simulink library "halin"  (R2021b)
settings: Solver=VariableStepAuto  StartTime=0.0  StopTime=10.0  RelTol=1e-3
undefined symbols (not defined in the file): KHAL_CAN1ABM1E2E_flg, KHAL_CAN1EPB1E2E_flg, KHAL_CAN1EPS1E2E_flg, KHAL_CAN1ESC1E2E_flg, KHAL_CAN1ESC5E2E_flg, KHAL_CAN3BMS1E2E_flg, KHAL_CAN3BMS6E2E_flg, KHAL_CAN3CCU1E2E_flg, KHAL_CAN3CCU2E2E_flg, KHAL_CAN3MCUNF1E2E_flg, KHAL_CAN3MCUNR1E2E_flg, KHAL_CAN3Shifter1E2E_flg, KHAL_CAN3Shifter2E2E_flg, KHAL_CAN6FCM2E2E_flg, KHAL_CAN6FCM4E2E_flg, TRUE
libraries: simulink x645, FVT_lib x212, hcu_lib x59
(part 9 of 23)

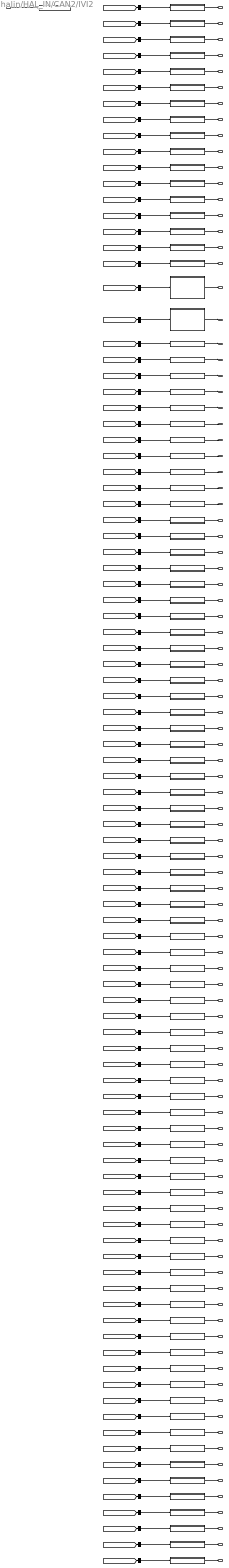
== system halin/HAL_IN/CAN2/IVI2 ==
  DT_CAN2_SG_IVI2 : Inport
  ACChgCurSet : Subsystem
  AVMErrSTA : Subsystem
  AVMOFFRecButt : Subsystem
  AVMParkingmode : Subsystem
  AVMparkingcancel : Subsystem
  AVMparkingexcute : Subsystem
  ApproachUnlockSW : Subsystem
  CAASSw : Subsystem
  CDLLockButt : Subsystem
  CDLUnlockButt : Subsystem
  DSEATantiset : Subsystem
  DSEATentryfunset : Subsystem
  DSEATventreq : Subsystem
  Distanceunit : Subsystem
  ESCSWCmd : Subsystem
  FSOffSw : Subsystem
  FollowMeSW : Subsystem
  GPSLAT : Subsystem
  GPSLONG : Subsystem
  HeadLampSW : Subsystem
  HoodLatchSW : Subsystem
  IVIACCAdaptiveSta : Subsystem
  IVIAirIntZ3Cmd : Subsystem
  IVIChargePortSWSta : Subsystem
  IVICreepSWReq : Subsystem
  IVIDSEATFroEdgeHeightCmd : Subsystem
  IVIDSEATHeaterCmd : Subsystem
  IVIDSEATHeightCmd : Subsystem
  IVIDSEATMemory1Sta : Subsystem
  IVIDSEATMemory2Sta : Subsystem
  IVIDSEATMemoryOPTCLSSta : Subsystem
  IVIDSEATReclineCmd : Subsystem
  IVIDSEATSlideCmd : Subsystem
  IVIFGSAirIntCmd : Subsystem
  IVIFGSChCmd : Subsystem
  IVIIONSWCmd : Subsystem
  IVIISAOffsetSpd : Subsystem
  IVINightModeSta : Subsystem
  IVIPSEATHeaterCmd : Subsystem
  IVIPSEATReclineCmd : Subsystem
  IVIPSEATSlideCmd : Subsystem
  IVIPTGModeSW : Subsystem
  IVIPTGOpenHeight : Subsystem
  IVIPTGStaSW : Subsystem
  IVIPTGUSStaSW : Subsystem
  IVIPWModeReq : Subsystem
  IVIPwrLockSW : Subsystem
  IVIPwroffreq : Subsystem
  IVIRRDefReq : Subsystem
  IVIReqV2L : Subsystem
  IVISWCRUndefinedSta : Subsystem
  IVIScreen : Subsystem
  IVIStartChgreq : Subsystem
  IVIStatus : Subsystem
  IVIStopChgreq : Subsystem
  IVITrailerCheckReqSta : Subsystem
  IVITrailerModeSWSta : Subsystem
  IVITriggerreq : Subsystem
  IVIUnlockChgreq : Subsystem
  IVIWIMAINSW : Subsystem
  LDrvControlCommand : Subsystem
  LPasControlCommand : Subsystem
  LRLDControlCommand : Subsystem
  LRRDControlCommand : Subsystem
  LightShowStartReq : Subsystem
  LightShowStopReq : Subsystem
  MFRDNBrightReq : Subsystem
  OFFACMODE : Subsystem
  PSEATventreq : Subsystem
  PerdV2L : Subsystem
  RFogLampSW : Subsystem
  RollModeSWCmd : Subsystem
  RoomLampMode : Subsystem
  SOCADJBUTT : Subsystem
  SOCLimitSet : Subsystem
  SOCV2LLimit : Subsystem
  SchedChgStart : Subsystem
  SchedChgStop : Subsystem
  SchedChgbutt : Subsystem
  SchedChglimit : Subsystem
  SchedChgwake : Subsystem
  SenstivityPosition : Subsystem
  SetUnlockSingle : Subsystem
  TCSSWCmd : Subsystem
  TPMSCaliButt : Subsystem
  TPMSResButt : Subsystem
  TurnSwTimeSet : Subsystem
  WalkawayLockSW : Subsystem
  WlcmLightMode : Subsystem
  bus_selector : BusSelector  OutputSignals=CAN2_AC_Chg_Cur_Set
  bus_selector1 : BusSelector  OutputSignals=CAN2_AVM_Err_STA
  bus_selector10 : BusSelector  OutputSignals=CAN2_DSEAT_anti_set
  bus_selector11 : BusSelector  OutputSignals=CAN2_DSEAT_entryfun_set
  bus_selector12 : BusSelector  OutputSignals=CAN2_DSEAT_vent_req
  bus_selector13 : BusSelector  OutputSignals=CAN2_Distance_unit
  bus_selector14 : BusSelector  OutputSignals=CAN2_ESC_SW_Cmd
  bus_selector15 : BusSelector  OutputSignals=CAN2_FS_Off_Sw
  bus_selector16 : BusSelector  OutputSignals=CAN2_FollowMeSW
  bus_selector17 : BusSelector  OutputSignals=CAN2_GPS_LAT
  bus_selector18 : BusSelector  OutputSignals=CAN2_GPS_LONG
  bus_selector19 : BusSelector  OutputSignals=CAN2_HeadLampSW
  bus_selector2 : BusSelector  OutputSignals=CAN2_AVM_OFF_Rec_Butt
  bus_selector20 : BusSelector  OutputSignals=CAN2_Hood_Latch_SW
  bus_selector21 : BusSelector  OutputSignals=CAN2_IVI_ACC_Adaptive_Sta
  bus_selector22 : BusSelector  OutputSignals=CAN2_IVI_AirIntZ3_Cmd
  bus_selector23 : BusSelector  OutputSignals=CAN2_IVI_ChargePortSW_Sta
  bus_selector24 : BusSelector  OutputSignals=CAN2_IVI_CreepSW_Req
  bus_selector25 : BusSelector  OutputSignals=CAN2_IVI_DSEATHeater_Cmd
  bus_selector26 : BusSelector  OutputSignals=CAN2_IVI_DSEAT_FroEdge_Height_Cmd
  bus_selector27 : BusSelector  OutputSignals=CAN2_IVI_DSEAT_Height_Cmd
  bus_selector28 : BusSelector  OutputSignals=CAN2_IVI_DSEAT_Memory1_Sta
  bus_selector29 : BusSelector  OutputSignals=CAN2_IVI_DSEAT_Memory2_Sta
  bus_selector3 : BusSelector  OutputSignals=CAN2_AVM_Parking_mode
  bus_selector30 : BusSelector  OutputSignals=CAN2_IVI_DSEAT_Memory_OPTCLS_Sta
  bus_selector31 : BusSelector  OutputSignals=CAN2_IVI_DSEAT_Recline_Cmd
  bus_selector32 : BusSelector  OutputSignals=CAN2_IVI_DSEAT_Slide_Cmd
  bus_selector33 : BusSelector  OutputSignals=CAN2_IVI_FGSAirInt_Cmd
  bus_selector34 : BusSelector  OutputSignals=CAN2_IVI_FGSCh_Cmd
  bus_selector35 : BusSelector  OutputSignals=CAN2_IVI_IONSW_Cmd
  bus_selector36 : BusSelector  OutputSignals=CAN2_IVI_ISA_OffsetSpd
  bus_selector37 : BusSelector  OutputSignals=CAN2_IVI_Night_Mode_Sta
  bus_selector38 : BusSelector  OutputSignals=CAN2_IVI_PSEATHeater_Cmd
  bus_selector39 : BusSelector  OutputSignals=CAN2_IVI_PSEAT_Recline_Cmd
  bus_selector4 : BusSelector  OutputSignals=CAN2_AVM_parking_cancel
  bus_selector40 : BusSelector  OutputSignals=CAN2_IVI_PSEAT_Slide_Cmd
  bus_selector41 : BusSelector  OutputSignals=CAN2_IVI_PTG_Mode_SW
  bus_selector42 : BusSelector  OutputSignals=CAN2_IVI_PTG_Open_Height
  bus_selector43 : BusSelector  OutputSignals=CAN2_IVI_PTG_Sta_SW
  bus_selector44 : BusSelector  OutputSignals=CAN2_IVI_PTG_USSta_SW
  bus_selector45 : BusSelector  OutputSignals=CAN2_IVI_PW_Mode_Req
  bus_selector46 : BusSelector  OutputSignals=CAN2_IVI_PwrLockSW
  bus_selector47 : BusSelector  OutputSignals=CAN2_IVI_Pwroff_req
  bus_selector48 : BusSelector  OutputSignals=CAN2_IVI_RR_Def_Req
  bus_selector49 : BusSelector  OutputSignals=CAN2_IVI_Req_V2L
  bus_selector5 : BusSelector  OutputSignals=CAN2_AVM_parking_excute
  bus_selector50 : BusSelector  OutputSignals=CAN2_IVI_SWC_RUndefined_Sta
  bus_selector51 : BusSelector  OutputSignals=CAN2_IVI_Screen
  bus_selector52 : BusSelector  OutputSignals=CAN2_IVI_Start_Chg_req
  bus_selector53 : BusSelector  OutputSignals=CAN2_IVI_Status
  bus_selector54 : BusSelector  OutputSignals=CAN2_IVI_Stop_Chg_req
  bus_selector55 : BusSelector  OutputSignals=CAN2_IVI_TrailerCheckReq_Sta
  bus_selector56 : BusSelector  OutputSignals=CAN2_IVI_TrailerModeSW_Sta
  bus_selector57 : BusSelector  OutputSignals=CAN2_IVI_Trigger_req
  bus_selector58 : BusSelector  OutputSignals=CAN2_IVI_Unlock_Chg_req
  bus_selector59 : BusSelector  OutputSignals=CAN2_IVI_WI_MAIN_SW
  bus_selector6 : BusSelector  OutputSignals=CAN2_Approach_Unlock_SW
  bus_selector60 : BusSelector  OutputSignals=CAN2_L_Drv_ControlCommand
  bus_selector61 : BusSelector  OutputSignals=CAN2_L_Pas_ControlCommand
  bus_selector62 : BusSelector  OutputSignals=CAN2_L_RLD_ControlCommand
  bus_selector63 : BusSelector  OutputSignals=CAN2_L_RRD_ControlCommand
  bus_selector64 : BusSelector  OutputSignals=CAN2_Light_ShowStart_Req
  bus_selector65 : BusSelector  OutputSignals=CAN2_Light_ShowStop_Req
  bus_selector66 : BusSelector  OutputSignals=CAN2_MFRD_N_Bright_Req
  bus_selector67 : BusSelector  OutputSignals=CAN2_OFF_AC_MODE
  bus_selector68 : BusSelector  OutputSignals=CAN2_PSEAT_vent_req
  bus_selector69 : BusSelector  OutputSignals=CAN2_Perd_V2L
  bus_selector7 : BusSelector  OutputSignals=CAN2_CAAS_Sw
  bus_selector70 : BusSelector  OutputSignals=CAN2_RFogLampSW
  bus_selector71 : BusSelector  OutputSignals=CAN2_Roll_Mode_SW_Cmd
  bus_selector72 : BusSelector  OutputSignals=CAN2_RoomLampMode
  bus_selector73 : BusSelector  OutputSignals=CAN2_SOC_ADJ_BUTT
  bus_selector74 : BusSelector  OutputSignals=CAN2_SOC_Limit_Set
  bus_selector75 : BusSelector  OutputSignals=CAN2_SOC_V2LLimit
  bus_selector76 : BusSelector  OutputSignals=CAN2_Sched_Chg_Start
  bus_selector77 : BusSelector  OutputSignals=CAN2_Sched_Chg_Stop
  bus_selector78 : BusSelector  OutputSignals=CAN2_Sched_Chg_butt
  bus_selector79 : BusSelector  OutputSignals=CAN2_Sched_Chg_limit
  bus_selector8 : BusSelector  OutputSignals=CAN2_CDL_Lock_Butt
  bus_selector80 : BusSelector  OutputSignals=CAN2_Sched_Chg_wake
  bus_selector81 : BusSelector  OutputSignals=CAN2_SenstivityPosition
  bus_selector82 : BusSelector  OutputSignals=CAN2_SetUnlockSingle
  bus_selector83 : BusSelector  OutputSignals=CAN2_TCS_SW_Cmd
  bus_selector84 : BusSelector  OutputSignals=CAN2_TPMS_Cali_Butt
  bus_selector85 : BusSelector  OutputSignals=CAN2_TPMS_Res_Butt
  bus_selector86 : BusSelector  OutputSignals=CAN2_TurnSwTimeSet
  bus_selector87 : BusSelector  OutputSignals=CAN2_Walkaway_Lock_SW
  bus_selector88 : BusSelector  OutputSignals=CAN2_WlcmLight_Mode
  bus_selector89 : BusSelector  OutputSignals=CAN2_sigAirIntenZon1Req
  bus_selector9 : BusSelector  OutputSignals=CAN2_CDL_Unlock_Butt
  bus_selector90 : BusSelector  OutputSignals=CAN2_sigDfrstReq
  bus_selector91 : BusSelector  OutputSignals=CAN2_sigFaceReq
  bus_selector92 : BusSelector  OutputSignals=CAN2_sigFootReq
  bus_selector93 : BusSelector  OutputSignals=CAN2_sigRecircReq
  bus_selector94 : BusSelector  OutputSignals=CAN2_sigSetTempZon1Req
  bus_selector95 : BusSelector  OutputSignals=CAN2_sigSetTempZon2Req
  sigAirIntenZon1Req : Subsystem
  sigDfrstReq : Subsystem
  sigFaceReq : Subsystem
  sigFootReq : Subsystem
  sigRecircReq : Subsystem
  sigSetTempZon1Req : Subsystem
  sigSetTempZon2Req : Subsystem
  VHAL_ACChgCurSet_A : Outport
  VHAL_AVMErrSTA_flg : Outport  Port=2
  VHAL_AVMOFFRecButt_flg : Outport  Port=3
  VHAL_AVMParkingmode_enum : Outport  Port=4
  VHAL_AVMparkingcancel_enum : Outport  Port=5
  VHAL_AVMparkingexcute_enum : Outport  Port=6
  VHAL_ApproachUnlockSW_flg : Outport  Port=7
  VHAL_CAASSw_enum : Outport  Port=8
  VHAL_CDLLockButt_flg : Outport  Port=9
  VHAL_CDLUnlockButt_flg : Outport  Port=10
  VHAL_DSEATantiset_flg : Outport  Port=11
  VHAL_DSEATentryfunset_flg : Outport  Port=12
  VHAL_DSEATventreq_enum : Outport  Port=13
  VHAL_Distanceunit_flg : Outport  Port=14
  VHAL_ESCSWCmd_enum : Outport  Port=15
  VHAL_FSOffSw_enum : Outport  Port=16
  VHAL_FollowMeSW_flg : Outport  Port=17
  VHAL_GPSLAT_s : Outport  Port=18
  VHAL_GPSLONG_enum : Outport  Port=19
  VHAL_HeadLampSW_enum : Outport  Port=20
  VHAL_HoodLatchSW_enum : Outport  Port=21
  VHAL_IVIACCAdaptiveSta_flg : Outport  Port=22
  VHAL_IVIAirIntZ3Cmd_enum : Outport  Port=23
  VHAL_IVIChargePortSWSta_flg : Outport  Port=24
  VHAL_IVICreepSWReq_flg : Outport  Port=25
  VHAL_IVIDSEATHeaterCmd_enum : Outport  Port=26
  VHAL_IVIDSEATFroEdgeHeightCmd_enum : Outport  Port=27
  VHAL_IVIDSEATHeightCmd_enum : Outport  Port=28
  VHAL_IVIDSEATMemory1Sta_flg : Outport  Port=29
  VHAL_IVIDSEATMemory2Sta_flg : Outport  Port=30
  VHAL_IVIDSEATMemoryOPTCLSSta_flg : Outport  Port=31
  VHAL_IVIDSEATReclineCmd_enum : Outport  Port=32
  VHAL_IVIDSEATSlideCmd_enum : Outport  Port=33
  VHAL_IVIFGSAirIntCmd_enum : Outport  Port=34
  VHAL_IVIFGSChCmd_enum : Outport  Port=35
  VHAL_IVIIONSWCmd_flg : Outport  Port=36
  VHAL_IVIISAOffsetSpd_enum : Outport  Port=37
  VHAL_IVINightModeSta_flg : Outport  Port=38
  VHAL_IVIPSEATHeaterCmd_enum : Outport  Port=39
  VHAL_IVIPSEATReclineCmd_enum : Outport  Port=40
  VHAL_IVIPSEATSlideCmd_enum : Outport  Port=41
  VHAL_IVIPTGModeSW_enum : Outport  Port=42
  VHAL_IVIPTGOpenHeight_enum : Outport  Port=43
  VHAL_IVIPTGStaSW_enum : Outport  Port=44
  VHAL_IVIPTGUSStaSW_flg : Outport  Port=45
  VHAL_IVIPWModeReq_enum : Outport  Port=46
  VHAL_IVIPwrLockSW_enum : Outport  Port=47
  VHAL_IVIPwroffreq_flg : Outport  Port=48
  VHAL_IVIRRDefReq_flg : Outport  Port=49
  VHAL_IVIReqV2L_enum : Outport  Port=50
  VHAL_IVISWCRUndefinedSta_enum : Outport  Port=51
  VHAL_IVIScreen_enum : Outport  Port=52
  VHAL_IVIStartChgreq_flg : Outport  Port=53
  VHAL_IVIStatus_flg : Outport  Port=54
  VHAL_IVIStopChgreq_flg : Outport  Port=55
  VHAL_IVITrailerCheckReqSta_flg : Outport  Port=56
  VHAL_IVITrailerModeSWSta_flg : Outport  Port=57
  VHAL_IVITriggerreq_flg : Outport  Port=58
  VHAL_IVIUnlockChgreq_flg : Outport  Port=59
  VHAL_IVIWIMAINSW_flg : Outport  Port=60
  VHAL_LDrvControlCommand_pct : Outport  Port=61
  VHAL_LPasControlCommand_pct : Outport  Port=62
  VHAL_LRLDControlCommand_pct : Outport  Port=63
  VHAL_LRRDControlCommand_pct : Outport  Port=64
  VHAL_LightShowStartReq_flg : Outport  Port=65
  VHAL_LightShowStopReq_flg : Outport  Port=66
  VHAL_MFRDNBrightReq_pct : Outport  Port=67
  VHAL_OFFACMODE_enum : Outport  Port=68
  VHAL_PSEATventreq_enum : Outport  Port=69
  VHAL_PerdV2L_enum : Outport  Port=70
  VHAL_RFogLampSW_flg : Outport  Port=71
  VHAL_RollModeSWCmd_enum : Outport  Port=72
  VHAL_RoomLampMode_flg : Outport  Port=73
  VHAL_SOCADJBUTT_flg : Outport  Port=74
  VHAL_SOCLimitSet_pct : Outport  Port=75
  VHAL_SOCV2LLimit_pct : Outport  Port=76
  VHAL_SchedChgStart_flg : Outport  Port=77
  VHAL_SchedChgStop_flg : Outport  Port=78
  VHAL_SchedChgbutt_flg : Outport  Port=79
  VHAL_SchedChglimit_pct : Outport  Port=80
  VHAL_SchedChgwake_flg : Outport  Port=81
  VHAL_SenstivityPosition_enum : Outport  Port=82
  VHAL_SetUnlockSingle_flg : Outport  Port=83
  VHAL_TCSSWCmd_enum : Outport  Port=84
  VHAL_TPMSCaliButt_flg : Outport  Port=85
  VHAL_TPMSResButt_flg : Outport  Port=86
  VHAL_TurnSwTimeSet_enum : Outport  Port=87
  VHAL_WalkawayLockSW_flg : Outport  Port=88
  VHAL_WlcmLightMode_enum : Outport  Port=89
  VHAL_sigAirIntenZon1Req_enum : Outport  Port=90
  VHAL_sigDfrstReq_flg : Outport  Port=91
  VHAL_sigFaceReq_flg : Outport  Port=92
  VHAL_sigFootReq_flg : Outport  Port=93
  VHAL_sigRecircReq_flg : Outport  Port=94
  VHAL_sigSetTempZon1Req_C : Outport  Port=95
  VHAL_sigSetTempZon2Req_C : Outport  Port=96
  wires:
  DT_CAN2_SG_IVI2/1 -> [DT_CAN2_SG_IVI2]
  [DT_CAN2_SG_IVI2] -> bus_selector/1
  bus_selector/1 -> ACChgCurSet/1(AC_Chg_Cur_Set)  "<CAN2_AC_Chg_Cur_Set>"
  ACChgCurSet/1(VHAL_ACChgCurSet_A) -> VHAL_ACChgCurSet_A/1
  [DT_CAN2_SG_IVI2] -> bus_selector1/1
  bus_selector1/1 -> AVMErrSTA/1(AVM_Err_STA)  "<CAN2_AVM_Err_STA>"
  AVMErrSTA/1(VHAL_AVMErrSTA_flg) -> VHAL_AVMErrSTA_flg/1
  [DT_CAN2_SG_IVI2] -> bus_selector2/1
  bus_selector2/1 -> AVMOFFRecButt/1(AVM_OFF_Rec_Butt)  "<CAN2_AVM_OFF_Rec_Butt>"
  AVMOFFRecButt/1(VHAL_AVMOFFRecButt_flg) -> VHAL_AVMOFFRecButt_flg/1
  [DT_CAN2_SG_IVI2] -> bus_selector3/1
  bus_selector3/1 -> AVMParkingmode/1(AVM_Parking_mode)  "<CAN2_AVM_Parking_mode>"
  AVMParkingmode/1(VHAL_AVMParkingmode_enum) -> VHAL_AVMParkingmode_enum/1
  [DT_CAN2_SG_IVI2] -> bus_selector4/1
  bus_selector4/1 -> AVMparkingcancel/1(AVM_parking_cancel)  "<CAN2_AVM_parking_cancel>"
  AVMparkingcancel/1(VHAL_AVMparkingcancel_enum) -> VHAL_AVMparkingcancel_enum/1
  [DT_CAN2_SG_IVI2] -> bus_selector5/1
  bus_selector5/1 -> AVMparkingexcute/1(AVM_parking_excute)  "<CAN2_AVM_parking_excute>"
  AVMparkingexcute/1(VHAL_AVMparkingexcute_enum) -> VHAL_AVMparkingexcute_enum/1
  [DT_CAN2_SG_IVI2] -> bus_selector6/1
  bus_selector6/1 -> ApproachUnlockSW/1(Approach_Unlock_SW)  "<CAN2_Approach_Unlock_SW>"
  ApproachUnlockSW/1(VHAL_ApproachUnlockSW_flg) -> VHAL_ApproachUnlockSW_flg/1
  [DT_CAN2_SG_IVI2] -> bus_selector7/1
  bus_selector7/1 -> CAASSw/1(CAAS_Sw)  "<CAN2_CAAS_Sw>"
  CAASSw/1(VHAL_CAASSw_enum) -> VHAL_CAASSw_enum/1
  [DT_CAN2_SG_IVI2] -> bus_selector8/1
  bus_selector8/1 -> CDLLockButt/1(CDL_Lock_Butt)  "<CAN2_CDL_Lock_Butt>"
  CDLLockButt/1(VHAL_CDLLockButt_flg) -> VHAL_CDLLockButt_flg/1
  [DT_CAN2_SG_IVI2] -> bus_selector9/1
  bus_selector9/1 -> CDLUnlockButt/1(CDL_Unlock_Butt)  "<CAN2_CDL_Unlock_Butt>"
  CDLUnlockButt/1(VHAL_CDLUnlockButt_flg) -> VHAL_CDLUnlockButt_flg/1
  [DT_CAN2_SG_IVI2] -> bus_selector10/1
  bus_selector10/1 -> DSEATantiset/1(DSEAT_anti_set)  "<CAN2_DSEAT_anti_set>"
  DSEATantiset/1(VHAL_DSEATantiset_flg) -> VHAL_DSEATantiset_flg/1
  [DT_CAN2_SG_IVI2] -> bus_selector11/1
  bus_selector11/1 -> DSEATentryfunset/1(DSEAT_entryfun_set)  "<CAN2_DSEAT_entryfun_set>"
  DSEATentryfunset/1(VHAL_DSEATentryfunset_flg) -> VHAL_DSEATentryfunset_flg/1
  [DT_CAN2_SG_IVI2] -> bus_selector12/1
  bus_selector12/1 -> DSEATventreq/1(DSEAT_vent_req)  "<CAN2_DSEAT_vent_req>"
  DSEATventreq/1(VHAL_DSEATventreq_enum) -> VHAL_DSEATventreq_enum/1
  [DT_CAN2_SG_IVI2] -> bus_selector13/1
  bus_selector13/1 -> Distanceunit/1(Distance_unit)  "<CAN2_Distance_unit>"
  Distanceunit/1(VHAL_Distanceunit_flg) -> VHAL_Distanceunit_flg/1
  [DT_CAN2_SG_IVI2] -> bus_selector14/1
  bus_selector14/1 -> ESCSWCmd/1(ESC_SW_Cmd)  "<CAN2_ESC_SW_Cmd>"
  ESCSWCmd/1(VHAL_ESCSWCmd_enum) -> VHAL_ESCSWCmd_enum/1
  [DT_CAN2_SG_IVI2] -> bus_selector15/1
  bus_selector15/1 -> FSOffSw/1(FS_Off_Sw)  "<CAN2_FS_Off_Sw>"
  FSOffSw/1(VHAL_FSOffSw_enum) -> VHAL_FSOffSw_enum/1
  [DT_CAN2_SG_IVI2] -> bus_selector16/1
  bus_selector16/1 -> FollowMeSW/1(FollowMeSW)  "<CAN2_FollowMeSW>"
  FollowMeSW/1(VHAL_FollowMeSW_flg) -> VHAL_FollowMeSW_flg/1
  [DT_CAN2_SG_IVI2] -> bus_selector17/1
  bus_selector17/1 -> GPSLAT/1(GPS_LAT)  "<CAN2_GPS_LAT>"
  GPSLAT/1(VHAL_GPSLAT_s) -> VHAL_GPSLAT_s/1
  [DT_CAN2_SG_IVI2] -> bus_selector18/1
  bus_selector18/1 -> GPSLONG/1(GPS_LONG)  "<CAN2_GPS_LONG>"
  GPSLONG/1(VHAL_GPSLONG_enum) -> VHAL_GPSLONG_enum/1
  [DT_CAN2_SG_IVI2] -> bus_selector19/1
  bus_selector19/1 -> HeadLampSW/1(HeadLampSW)  "<CAN2_HeadLampSW>"
  HeadLampSW/1(VHAL_HeadLampSW_enum) -> VHAL_HeadLampSW_enum/1
  [DT_CAN2_SG_IVI2] -> bus_selector20/1
  bus_selector20/1 -> HoodLatchSW/1(Hood_Latch_SW)  "<CAN2_Hood_Latch_SW>"
  HoodLatchSW/1(VHAL_HoodLatchSW_enum) -> VHAL_HoodLatchSW_enum/1
  [DT_CAN2_SG_IVI2] -> bus_selector21/1
  bus_selector21/1 -> IVIACCAdaptiveSta/1(IVI_ACC_Adaptive_Sta)  "<CAN2_IVI_ACC_Adaptive_Sta>"
  IVIACCAdaptiveSta/1(VHAL_IVIACCAdaptiveSta_flg) -> VHAL_IVIACCAdaptiveSta_flg/1
  [DT_CAN2_SG_IVI2] -> bus_selector22/1
  bus_selector22/1 -> IVIAirIntZ3Cmd/1(IVI_AirIntZ3_Cmd)  "<CAN2_IVI_AirIntZ3_Cmd>"
  IVIAirIntZ3Cmd/1(VHAL_IVIAirIntZ3Cmd_enum) -> VHAL_IVIAirIntZ3Cmd_enum/1
  [DT_CAN2_SG_IVI2] -> bus_selector23/1
  bus_selector23/1 -> IVIChargePortSWSta/1(IVI_ChargePortSW_Sta)  "<CAN2_IVI_ChargePortSW_Sta>"
  IVIChargePortSWSta/1(VHAL_IVIChargePortSWSta_flg) -> VHAL_IVIChargePortSWSta_flg/1
  [DT_CAN2_SG_IVI2] -> bus_selector24/1
  bus_selector24/1 -> IVICreepSWReq/1(IVI_CreepSW_Req)  "<CAN2_IVI_CreepSW_Req>"
  IVICreepSWReq/1(VHAL_IVICreepSWReq_flg) -> VHAL_IVICreepSWReq_flg/1
  [DT_CAN2_SG_IVI2] -> bus_selector25/1
  bus_selector25/1 -> IVIDSEATHeaterCmd/1(IVI_DSEATHeater_Cmd)  "<CAN2_IVI_DSEATHeater_Cmd>"
  IVIDSEATHeaterCmd/1(VHAL_IVIDSEATHeaterCmd_enum) -> VHAL_IVIDSEATHeaterCmd_enum/1
  [DT_CAN2_SG_IVI2] -> bus_selector26/1
  bus_selector26/1 -> IVIDSEATFroEdgeHeightCmd/1(IVI_DSEAT_FroEdge_Height_Cmd)  "<CAN2_IVI_DSEAT_FroEdge_Height_Cmd>"
  IVIDSEATFroEdgeHeightCmd/1(VHAL_IVIDSEATFroEdgeHeightCmd_enum) -> VHAL_IVIDSEATFroEdgeHeightCmd_enum/1
  [DT_CAN2_SG_IVI2] -> bus_selector27/1
  bus_selector27/1 -> IVIDSEATHeightCmd/1(IVI_DSEAT_Height_Cmd)  "<CAN2_IVI_DSEAT_Height_Cmd>"
  IVIDSEATHeightCmd/1(VHAL_IVIDSEATHeightCmd_enum) -> VHAL_IVIDSEATHeightCmd_enum/1
  [DT_CAN2_SG_IVI2] -> bus_selector28/1
  bus_selector28/1 -> IVIDSEATMemory1Sta/1(IVI_DSEAT_Memory1_Sta)  "<CAN2_IVI_DSEAT_Memory1_Sta>"
  IVIDSEATMemory1Sta/1(VHAL_IVIDSEATMemory1Sta_flg) -> VHAL_IVIDSEATMemory1Sta_flg/1
  [DT_CAN2_SG_IVI2] -> bus_selector29/1
  bus_selector29/1 -> IVIDSEATMemory2Sta/1(IVI_DSEAT_Memory2_Sta)  "<CAN2_IVI_DSEAT_Memory2_Sta>"
  IVIDSEATMemory2Sta/1(VHAL_IVIDSEATMemory2Sta_flg) -> VHAL_IVIDSEATMemory2Sta_flg/1
  [DT_CAN2_SG_IVI2] -> bus_selector30/1
  bus_selector30/1 -> IVIDSEATMemoryOPTCLSSta/1(IVI_DSEAT_Memory_OPTCLS_Sta)  "<CAN2_IVI_DSEAT_Memory_OPTCLS_Sta>"
  IVIDSEATMemoryOPTCLSSta/1(VHAL_IVIDSEATMemoryOPTCLSSta_flg) -> VHAL_IVIDSEATMemoryOPTCLSSta_flg/1
  [DT_CAN2_SG_IVI2] -> bus_selector31/1
  bus_selector31/1 -> IVIDSEATReclineCmd/1(IVI_DSEAT_Recline_Cmd)  "<CAN2_IVI_DSEAT_Recline_Cmd>"
  IVIDSEATReclineCmd/1(VHAL_IVIDSEATReclineCmd_enum) -> VHAL_IVIDSEATReclineCmd_enum/1
  [DT_CAN2_SG_IVI2] -> bus_selector32/1
  bus_selector32/1 -> IVIDSEATSlideCmd/1(IVI_DSEAT_Slide_Cmd)  "<CAN2_IVI_DSEAT_Slide_Cmd>"
  IVIDSEATSlideCmd/1(VHAL_IVIDSEATSlideCmd_enum) -> VHAL_IVIDSEATSlideCmd_enum/1
  [DT_CAN2_SG_IVI2] -> bus_selector33/1
  bus_selector33/1 -> IVIFGSAirIntCmd/1(IVI_FGSAirInt_Cmd)  "<CAN2_IVI_FGSAirInt_Cmd>"
  IVIFGSAirIntCmd/1(VHAL_IVIFGSAirIntCmd_enum) -> VHAL_IVIFGSAirIntCmd_enum/1
  [DT_CAN2_SG_IVI2] -> bus_selector34/1
  bus_selector34/1 -> IVIFGSChCmd/1(IVI_FGSCh_Cmd)  "<CAN2_IVI_FGSCh_Cmd>"
  IVIFGSChCmd/1(VHAL_IVIFGSChCmd_enum) -> VHAL_IVIFGSChCmd_enum/1
  [DT_CAN2_SG_IVI2] -> bus_selector35/1
  bus_selector35/1 -> IVIIONSWCmd/1(IVI_IONSW_Cmd)  "<CAN2_IVI_IONSW_Cmd>"
  IVIIONSWCmd/1(VHAL_IVIIONSWCmd_flg) -> VHAL_IVIIONSWCmd_flg/1
  [DT_CAN2_SG_IVI2] -> bus_selector36/1
  bus_selector36/1 -> IVIISAOffsetSpd/1(IVI_ISA_OffsetSpd)  "<CAN2_IVI_ISA_OffsetSpd>"
  IVIISAOffsetSpd/1(VHAL_IVIISAOffsetSpd_enum) -> VHAL_IVIISAOffsetSpd_enum/1
  [DT_CAN2_SG_IVI2] -> bus_selector37/1
  bus_selector37/1 -> IVINightModeSta/1(IVI_Night_Mode_Sta)  "<CAN2_IVI_Night_Mode_Sta>"
  IVINightModeSta/1(VHAL_IVINightModeSta_flg) -> VHAL_IVINightModeSta_flg/1
  [DT_CAN2_SG_IVI2] -> bus_selector38/1
  bus_selector38/1 -> IVIPSEATHeaterCmd/1(IVI_PSEATHeater_Cmd)  "<CAN2_IVI_PSEATHeater_Cmd>"
  IVIPSEATHeaterCmd/1(VHAL_IVIPSEATHeaterCmd_enum) -> VHAL_IVIPSEATHeaterCmd_enum/1
  [DT_CAN2_SG_IVI2] -> bus_selector39/1
  bus_selector39/1 -> IVIPSEATReclineCmd/1(IVI_PSEAT_Recline_Cmd)  "<CAN2_IVI_PSEAT_Recline_Cmd>"
  IVIPSEATReclineCmd/1(VHAL_IVIPSEATReclineCmd_enum) -> VHAL_IVIPSEATReclineCmd_enum/1
  [DT_CAN2_SG_IVI2] -> bus_selector40/1
  bus_selector40/1 -> IVIPSEATSlideCmd/1(IVI_PSEAT_Slide_Cmd)  "<CAN2_IVI_PSEAT_Slide_Cmd>"
  IVIPSEATSlideCmd/1(VHAL_IVIPSEATSlideCmd_enum) -> VHAL_IVIPSEATSlideCmd_enum/1
  [DT_CAN2_SG_IVI2] -> bus_selector41/1
  bus_selector41/1 -> IVIPTGModeSW/1(IVI_PTG_Mode_SW)  "<CAN2_IVI_PTG_Mode_SW>"
  IVIPTGModeSW/1(VHAL_IVIPTGModeSW_enum) -> VHAL_IVIPTGModeSW_enum/1
  [DT_CAN2_SG_IVI2] -> bus_selector42/1
  bus_selector42/1 -> IVIPTGOpenHeight/1(IVI_PTG_Open_Height)  "<CAN2_IVI_PTG_Open_Height>"
  IVIPTGOpenHeight/1(VHAL_IVIPTGOpenHeight_enum) -> VHAL_IVIPTGOpenHeight_enum/1
  [DT_CAN2_SG_IVI2] -> bus_selector43/1
  bus_selector43/1 -> IVIPTGStaSW/1(IVI_PTG_Sta_SW)  "<CAN2_IVI_PTG_Sta_SW>"
  IVIPTGStaSW/1(VHAL_IVIPTGStaSW_enum) -> VHAL_IVIPTGStaSW_enum/1
  [DT_CAN2_SG_IVI2] -> bus_selector44/1
  bus_selector44/1 -> IVIPTGUSStaSW/1(IVI_PTG_USSta_SW)  "<CAN2_IVI_PTG_USSta_SW>"
  IVIPTGUSStaSW/1(VHAL_IVIPTGUSStaSW_flg) -> VHAL_IVIPTGUSStaSW_flg/1
  [DT_CAN2_SG_IVI2] -> bus_selector45/1
  bus_selector45/1 -> IVIPWModeReq/1(IVI_PW_Mode_Req)  "<CAN2_IVI_PW_Mode_Req>"
  IVIPWModeReq/1(VHAL_IVIPWModeReq_enum) -> VHAL_IVIPWModeReq_enum/1
  [DT_CAN2_SG_IVI2] -> bus_selector46/1
  bus_selector46/1 -> IVIPwrLockSW/1(IVI_PwrLockSW)  "<CAN2_IVI_PwrLockSW>"
  IVIPwrLockSW/1(VHAL_IVIPwrLockSW_enum) -> VHAL_IVIPwrLockSW_enum/1
  [DT_CAN2_SG_IVI2] -> bus_selector47/1
  bus_selector47/1 -> IVIPwroffreq/1(IVI_Pwroff_req)  "<CAN2_IVI_Pwroff_req>"
  IVIPwroffreq/1(VHAL_IVIPwroffreq_flg) -> VHAL_IVIPwroffreq_flg/1
  [DT_CAN2_SG_IVI2] -> bus_selector48/1
  bus_selector48/1 -> IVIRRDefReq/1(IVI_RR_Def_Req)  "<CAN2_IVI_RR_Def_Req>"
  IVIRRDefReq/1(VHAL_IVIRRDefReq_flg) -> VHAL_IVIRRDefReq_flg/1
  [DT_CAN2_SG_IVI2] -> bus_selector49/1
  bus_selector49/1 -> IVIReqV2L/1(IVI_Req_V2L)  "<CAN2_IVI_Req_V2L>"
  IVIReqV2L/1(VHAL_IVIReqV2L_enum) -> VHAL_IVIReqV2L_enum/1
  [DT_CAN2_SG_IVI2] -> bus_selector50/1
  bus_selector50/1 -> IVISWCRUndefinedSta/1(IVI_SWC_RUndefined_Sta)  "<CAN2_IVI_SWC_RUndefined_Sta>"
  IVISWCRUndefinedSta/1(VHAL_IVISWCRUndefinedSta_enum) -> VHAL_IVISWCRUndefinedSta_enum/1
  [DT_CAN2_SG_IVI2] -> bus_selector51/1
  bus_selector51/1 -> IVIScreen/1(IVI_Screen)  "<CAN2_IVI_Screen>"
  IVIScreen/1(VHAL_IVIScreen_enum) -> VHAL_IVIScreen_enum/1
  [DT_CAN2_SG_IVI2] -> bus_selector52/1
  bus_selector52/1 -> IVIStartChgreq/1(IVI_Start_Chg_req)  "<CAN2_IVI_Start_Chg_req>"
  IVIStartChgreq/1(VHAL_IVIStartChgreq_flg) -> VHAL_IVIStartChgreq_flg/1
  [DT_CAN2_SG_IVI2] -> bus_selector53/1
  bus_selector53/1 -> IVIStatus/1(IVI_Status)  "<CAN2_IVI_Status>"
  IVIStatus/1(VHAL_IVIStatus_flg) -> VHAL_IVIStatus_flg/1
  [DT_CAN2_SG_IVI2] -> bus_selector54/1
  bus_selector54/1 -> IVIStopChgreq/1(IVI_Stop_Chg_req)  "<CAN2_IVI_Stop_Chg_req>"
  IVIStopChgreq/1(VHAL_IVIStopChgreq_flg) -> VHAL_IVIStopChgreq_flg/1
  [DT_CAN2_SG_IVI2] -> bus_selector55/1
  bus_selector55/1 -> IVITrailerCheckReqSta/1(IVI_TrailerCheckReq_Sta)  "<CAN2_IVI_TrailerCheckReq_Sta>"
  IVITrailerCheckReqSta/1(VHAL_IVITrailerCheckReqSta_flg) -> VHAL_IVITrailerCheckReqSta_flg/1
  [DT_CAN2_SG_IVI2] -> bus_selector56/1
  bus_selector56/1 -> IVITrailerModeSWSta/1(IVI_TrailerModeSW_Sta)  "<CAN2_IVI_TrailerModeSW_Sta>"
  IVITrailerModeSWSta/1(VHAL_IVITrailerModeSWSta_flg) -> VHAL_IVITrailerModeSWSta_flg/1
  [DT_CAN2_SG_IVI2] -> bus_selector57/1
  bus_selector57/1 -> IVITriggerreq/1(IVI_Trigger_req)  "<CAN2_IVI_Trigger_req>"
  IVITriggerreq/1(VHAL_IVITriggerreq_flg) -> VHAL_IVITriggerreq_flg/1
  [DT_CAN2_SG_IVI2] -> bus_selector58/1
  bus_selector58/1 -> IVIUnlockChgreq/1(IVI_Unlock_Chg_req)  "<CAN2_IVI_Unlock_Chg_req>"
  IVIUnlockChgreq/1(VHAL_IVIUnlockChgreq_flg) -> VHAL_IVIUnlockChgreq_flg/1
  [DT_CAN2_SG_IVI2] -> bus_selector59/1
  bus_selector59/1 -> IVIWIMAINSW/1(IVI_WI_MAIN_SW)  "<CAN2_IVI_WI_MAIN_SW>"
  IVIWIMAINSW/1(VHAL_IVIWIMAINSW_flg) -> VHAL_IVIWIMAINSW_flg/1
  [DT_CAN2_SG_IVI2] -> bus_selector60/1
  bus_selector60/1 -> LDrvControlCommand/1(L_Drv_ControlCommand)  "<CAN2_L_Drv_ControlCommand>"
  LDrvControlCommand/1(VHAL_LDrvControlCommand_pct) -> VHAL_LDrvControlCommand_pct/1
  [DT_CAN2_SG_IVI2] -> bus_selector61/1
  bus_selector61/1 -> LPasControlCommand/1(L_Pas_ControlCommand)  "<CAN2_L_Pas_ControlCommand>"
  LPasControlCommand/1(VHAL_LPasControlCommand_pct) -> VHAL_LPasControlCommand_pct/1
  [DT_CAN2_SG_IVI2] -> bus_selector62/1
  bus_selector62/1 -> LRLDControlCommand/1(L_RLD_ControlCommand)  "<CAN2_L_RLD_ControlCommand>"
  LRLDControlCommand/1(VHAL_LRLDControlCommand_pct) -> VHAL_LRLDControlCommand_pct/1
  [DT_CAN2_SG_IVI2] -> bus_selector63/1
  bus_selector63/1 -> LRRDControlCommand/1(L_RRD_ControlCommand)  "<CAN2_L_RRD_ControlCommand>"
  LRRDControlCommand/1(VHAL_LRRDControlCommand_pct) -> VHAL_LRRDControlCommand_pct/1
  [DT_CAN2_SG_IVI2] -> bus_selector64/1
  bus_selector64/1 -> LightShowStartReq/1(Light_ShowStart_Req)  "<CAN2_Light_ShowStart_Req>"
  LightShowStartReq/1(VHAL_LightShowStartReq_flg) -> VHAL_LightShowStartReq_flg/1
  [DT_CAN2_SG_IVI2] -> bus_selector65/1
  bus_selector65/1 -> LightShowStopReq/1(Light_ShowStop_Req)  "<CAN2_Light_ShowStop_Req>"
  LightShowStopReq/1(VHAL_LightShowStopReq_flg) -> VHAL_LightShowStopReq_flg/1
  [DT_CAN2_SG_IVI2] -> bus_selector66/1
  bus_selector66/1 -> MFRDNBrightReq/1(MFRD_N_Bright_Req)  "<CAN2_MFRD_N_Bright_Req>"
  MFRDNBrightReq/1(VHAL_MFRDNBrightReq_pct) -> VHAL_MFRDNBrightReq_pct/1
  [DT_CAN2_SG_IVI2] -> bus_selector67/1
  bus_selector67/1 -> OFFACMODE/1(OFF_AC_MODE)  "<CAN2_OFF_AC_MODE>"
  OFFACMODE/1(VHAL_OFFACMODE_enum) -> VHAL_OFFACMODE_enum/1
  [DT_CAN2_SG_IVI2] -> bus_selector68/1
  bus_selector68/1 -> PSEATventreq/1(PSEAT_vent_req)  "<CAN2_PSEAT_vent_req>"
  PSEATventreq/1(VHAL_PSEATventreq_enum) -> VHAL_PSEATventreq_enum/1
  [DT_CAN2_SG_IVI2] -> bus_selector69/1
  bus_selector69/1 -> PerdV2L/1(Perd_V2L)  "<CAN2_Perd_V2L>"
  PerdV2L/1(VHAL_PerdV2L_enum) -> VHAL_PerdV2L_enum/1
  [DT_CAN2_SG_IVI2] -> bus_selector70/1
  bus_selector70/1 -> RFogLampSW/1(RFogLampSW)  "<CAN2_RFogLampSW>"
  RFogLampSW/1(VHAL_RFogLampSW_flg) -> VHAL_RFogLampSW_flg/1
  [DT_CAN2_SG_IVI2] -> bus_selector71/1
  bus_selector71/1 -> RollModeSWCmd/1(Roll_Mode_SW_Cmd)  "<CAN2_Roll_Mode_SW_Cmd>"
  RollModeSWCmd/1(VHAL_RollModeSWCmd_enum) -> VHAL_RollModeSWCmd_enum/1
  [DT_CAN2_SG_IVI2] -> bus_selector72/1
  bus_selector72/1 -> RoomLampMode/1(RoomLampMode)  "<CAN2_RoomLampMode>"
  RoomLampMode/1(VHAL_RoomLampMode_flg) -> VHAL_RoomLampMode_flg/1
  [DT_CAN2_SG_IVI2] -> bus_selector73/1
  bus_selector73/1 -> SOCADJBUTT/1(SOC_ADJ_BUTT)  "<CAN2_SOC_ADJ_BUTT>"
  SOCADJBUTT/1(VHAL_SOCADJBUTT_flg) -> VHAL_SOCADJBUTT_flg/1
  [DT_CAN2_SG_IVI2] -> bus_selector74/1
  bus_selector74/1 -> SOCLimitSet/1(SOC_Limit_Set)  "<CAN2_SOC_Limit_Set>"
  SOCLimitSet/1(VHAL_SOCLimitSet_pct) -> VHAL_SOCLimitSet_pct/1
  [DT_CAN2_SG_IVI2] -> bus_selector75/1
  bus_selector75/1 -> SOCV2LLimit/1(SOC_V2LLimit)  "<CAN2_SOC_V2LLimit>"
  SOCV2LLimit/1(VHAL_SOCV2LLimit_pct) -> VHAL_SOCV2LLimit_pct/1
  [DT_CAN2_SG_IVI2] -> bus_selector76/1
  bus_selector76/1 -> SchedChgStart/1(Sched_Chg_Start)  "<CAN2_Sched_Chg_Start>"
  SchedChgStart/1(VHAL_SchedChgStart_flg) -> VHAL_SchedChgStart_flg/1
  [DT_CAN2_SG_IVI2] -> bus_selector77/1
  bus_selector77/1 -> SchedChgStop/1(Sched_Chg_Stop)  "<CAN2_Sched_Chg_Stop>"
  SchedChgStop/1(VHAL_SchedChgStop_flg) -> VHAL_SchedChgStop_flg/1
  [DT_CAN2_SG_IVI2] -> bus_selector78/1
  bus_selector78/1 -> SchedChgbutt/1(Sched_Chg_butt)  "<CAN2_Sched_Chg_butt>"
  SchedChgbutt/1(VHAL_SchedChgbutt_flg) -> VHAL_SchedChgbutt_flg/1
  [DT_CAN2_SG_IVI2] -> bus_selector79/1
  bus_selector79/1 -> SchedChglimit/1(Sched_Chg_limit)  "<CAN2_Sched_Chg_limit>"
  SchedChglimit/1(VHAL_SchedChglimit_pct) -> VHAL_SchedChglimit_pct/1
  [DT_CAN2_SG_IVI2] -> bus_selector80/1
  bus_selector80/1 -> SchedChgwake/1(Sched_Chg_wake)  "<CAN2_Sched_Chg_wake>"
  SchedChgwake/1(VHAL_SchedChgwake_flg) -> VHAL_SchedChgwake_flg/1
  [DT_CAN2_SG_IVI2] -> bus_selector81/1
  bus_selector81/1 -> SenstivityPosition/1(SenstivityPosition)  "<CAN2_SenstivityPosition>"
  SenstivityPosition/1(VHAL_SenstivityPosition_enum) -> VHAL_SenstivityPosition_enum/1
  [DT_CAN2_SG_IVI2] -> bus_selector82/1
  bus_selector82/1 -> SetUnlockSingle/1(SetUnlockSingle)  "<CAN2_SetUnlockSingle>"
  SetUnlockSingle/1(VHAL_SetUnlockSingle_flg) -> VHAL_SetUnlockSingle_flg/1
  [DT_CAN2_SG_IVI2] -> bus_selector83/1
  bus_selector83/1 -> TCSSWCmd/1(TCS_SW_Cmd)  "<CAN2_TCS_SW_Cmd>"
  TCSSWCmd/1(VHAL_TCSSWCmd_enum) -> VHAL_TCSSWCmd_enum/1
  [DT_CAN2_SG_IVI2] -> bus_selector84/1
  bus_selector84/1 -> TPMSCaliButt/1(TPMS_Cali_Butt)  "<CAN2_TPMS_Cali_Butt>"
  TPMSCaliButt/1(VHAL_TPMSCaliButt_flg) -> VHAL_TPMSCaliButt_flg/1
  [DT_CAN2_SG_IVI2] -> bus_selector85/1
  bus_selector85/1 -> TPMSResButt/1(TPMS_Res_Butt)  "<CAN2_TPMS_Res_Butt>"
  TPMSResButt/1(VHAL_TPMSResButt_flg) -> VHAL_TPMSResButt_flg/1
  [DT_CAN2_SG_IVI2] -> bus_selector86/1
  bus_selector86/1 -> TurnSwTimeSet/1(TurnSwTimeSet)  "<CAN2_TurnSwTimeSet>"
  TurnSwTimeSet/1(VHAL_TurnSwTimeSet_enum) -> VHAL_TurnSwTimeSet_enum/1
  [DT_CAN2_SG_IVI2] -> bus_selector87/1
  bus_selector87/1 -> WalkawayLockSW/1(Walkaway_Lock_SW)  "<CAN2_Walkaway_Lock_SW>"
  WalkawayLockSW/1(VHAL_WalkawayLockSW_flg) -> VHAL_WalkawayLockSW_flg/1
  [DT_CAN2_SG_IVI2] -> bus_selector88/1
  bus_selector88/1 -> WlcmLightMode/1(WlcmLight_Mode)  "<CAN2_WlcmLight_Mode>"
  WlcmLightMode/1(VHAL_WlcmLightMode_enum) -> VHAL_WlcmLightMode_enum/1
  [DT_CAN2_SG_IVI2] -> bus_selector89/1
  bus_selector89/1 -> sigAirIntenZon1Req/1(sigAirIntenZon1Req)  "<CAN2_sigAirIntenZon1Req>"
  sigAirIntenZon1Req/1(VHAL_sigAirIntenZon1Req_enum) -> VHAL_sigAirIntenZon1Req_enum/1
  [DT_CAN2_SG_IVI2] -> bus_selector90/1
  bus_selector90/1 -> sigDfrstReq/1(sigDfrstReq)  "<CAN2_sigDfrstReq>"
  sigDfrstReq/1(VHAL_sigDfrstReq_flg) -> VHAL_sigDfrstReq_flg/1
  [DT_CAN2_SG_IVI2] -> bus_selector91/1
  bus_selector91/1 -> sigFaceReq/1(sigFaceReq)  "<CAN2_sigFaceReq>"
  sigFaceReq/1(VHAL_sigFaceReq_flg) -> VHAL_sigFaceReq_flg/1
  [DT_CAN2_SG_IVI2] -> bus_selector92/1
  bus_selector92/1 -> sigFootReq/1(sigFootReq)  "<CAN2_sigFootReq>"
  sigFootReq/1(VHAL_sigFootReq_flg) -> VHAL_sigFootReq_flg/1
  [DT_CAN2_SG_IVI2] -> bus_selector93/1
  bus_selector93/1 -> sigRecircReq/1(sigRecircReq)  "<CAN2_sigRecircReq>"
  sigRecircReq/1(VHAL_sigRecircReq_flg) -> VHAL_sigRecircReq_flg/1
  [DT_CAN2_SG_IVI2] -> bus_selector94/1
  bus_selector94/1 -> sigSetTempZon1Req/1(sigSetTempZon1Req)  "<CAN2_sigSetTempZon1Req>"
  sigSetTempZon1Req/1(VHAL_sigSetTempZon1Req_C) -> VHAL_sigSetTempZon1Req_C/1
  [DT_CAN2_SG_IVI2] -> bus_selector95/1
  bus_selector95/1 -> sigSetTempZon2Req/1(sigSetTempZon2Req)  "<CAN2_sigSetTempZon2Req>"
  sigSetTempZon2Req/1(VHAL_sigSetTempZon2Req_C) -> VHAL_sigSetTempZon2Req_C/1

== system halin/HAL_IN/CAN2/IVI3 ==
  DT_CAN2_SG_IVI3 : Inport
  IVICLBlowerYSta : Subsystem
  IVICLBlowerZSta : Subsystem
  IVICRBlowerYSta : Subsystem
  IVICRBlowerZSta : Subsystem
  IVIDrBlowerModeSta : Subsystem
  IVIDrBlowerYSta : Subsystem
  IVIDrBlowerZSta : Subsystem
  IVIHMICustmiFunSta : Subsystem
  IVIHMICustmiKEYSta : Subsystem
  IVILSEATventCmd : Subsystem
  IVIMLFMostCmd : Subsystem
  IVIMLFootLiftCmd : Subsystem
  IVIMLNapModeCmd : Subsystem
  IVIMLReclinerCmd : Subsystem
  IVIMLRestoreCmd : Subsystem
  IVIMLSEATventCmd : Subsystem
  IVIMLSeatLiftCmd : Subsystem
  IVIMLSldRestoreCmd : Subsystem
  IVIMLSliderCmd : Subsystem
  IVIMLZeroGravityCmd : Subsystem
  IVIMRFMostCmd : Subsystem
  IVIMRFootLiftCmd : Subsystem
  IVIMRNapModeCmd : Subsystem
  IVIMRReclinerCmd : Subsystem
  IVIMRRestoreCmd : Subsystem
  IVIMRSEATventCmd : Subsystem
  IVIMRSeatLiftCmd : Subsystem
  IVIMRSldRestoreCmd : Subsystem
  IVIMRSliderCmd : Subsystem
  IVIMRZeroGravityCmd : Subsystem
  IVIPsBlowerModeSta : Subsystem
  IVIPsBlowerYSta : Subsystem
  IVIPsBlowerZSta : Subsystem
  IVIRSEATventCmd : Subsystem
  IVISnowModeCmd : Subsystem
  IVIUserTakeOverAPSSta : Subsystem
  IVIZon1WindDirSWReqSta : Subsystem
  bus_selector : BusSelector  OutputSignals=CAN2_IVI_CLBlower_Y_Sta
  bus_selector1 : BusSelector  OutputSignals=CAN2_IVI_CLBlower_Z_Sta
  bus_selector10 : BusSelector  OutputSignals=CAN2_IVI_MLFMost_Cmd
  bus_selector11 : BusSelector  OutputSignals=CAN2_IVI_MLFootLift_Cmd
  bus_selector12 : BusSelector  OutputSignals=CAN2_IVI_MLNapMode_Cmd
  bus_selector13 : BusSelector  OutputSignals=CAN2_IVI_MLRecliner_Cmd
  bus_selector14 : BusSelector  OutputSignals=CAN2_IVI_MLRestore_Cmd
  bus_selector15 : BusSelector  OutputSignals=CAN2_IVI_MLSEATvent_Cmd
  bus_selector16 : BusSelector  OutputSignals=CAN2_IVI_MLSeatLift_Cmd
  bus_selector17 : BusSelector  OutputSignals=CAN2_IVI_MLSldRestore_Cmd
  bus_selector18 : BusSelector  OutputSignals=CAN2_IVI_MLSlider_Cmd
  bus_selector19 : BusSelector  OutputSignals=CAN2_IVI_MLZeroGravity_Cmd
  bus_selector2 : BusSelector  OutputSignals=CAN2_IVI_CRBlower_Y_Sta
  bus_selector20 : BusSelector  OutputSignals=CAN2_IVI_MRFMost_Cmd
  bus_selector21 : BusSelector  OutputSignals=CAN2_IVI_MRFootLift_Cmd
  bus_selector22 : BusSelector  OutputSignals=CAN2_IVI_MRNapMode_Cmd
  bus_selector23 : BusSelector  OutputSignals=CAN2_IVI_MRRecliner_Cmd
  bus_selector24 : BusSelector  OutputSignals=CAN2_IVI_MRRestore_Cmd
  bus_selector25 : BusSelector  OutputSignals=CAN2_IVI_MRSEATvent_Cmd
  bus_selector26 : BusSelector  OutputSignals=CAN2_IVI_MRSeatLift_Cmd
  bus_selector27 : BusSelector  OutputSignals=CAN2_IVI_MRSldRestore_Cmd
  bus_selector28 : BusSelector  OutputSignals=CAN2_IVI_MRSlider_Cmd
  bus_selector29 : BusSelector  OutputSignals=CAN2_IVI_MRZeroGravity_Cmd
  bus_selector3 : BusSelector  OutputSignals=CAN2_IVI_CRBlower_Z_Sta
  bus_selector30 : BusSelector  OutputSignals=CAN2_IVI_PsBlower_Mode_Sta
  bus_selector31 : BusSelector  OutputSignals=CAN2_IVI_PsBlower_Y_Sta
  bus_selector32 : BusSelector  OutputSignals=CAN2_IVI_PsBlower_Z_Sta
  bus_selector33 : BusSelector  OutputSignals=CAN2_IVI_RSEATvent_Cmd
  bus_selector34 : BusSelector  OutputSignals=CAN2_IVI_SnowMode_Cmd
  bus_selector35 : BusSelector  OutputSignals=CAN2_IVI_UserTakeOver_APS_Sta
  bus_selector36 : BusSelector  OutputSignals=CAN2_IVI_Zon1WindDirSWReq_Sta
  bus_selector4 : BusSelector  OutputSignals=CAN2_IVI_DrBlower_Mode_Sta
  bus_selector5 : BusSelector  OutputSignals=CAN2_IVI_DrBlower_Y_Sta
  bus_selector6 : BusSelector  OutputSignals=CAN2_IVI_DrBlower_Z_Sta
  bus_selector7 : BusSelector  OutputSignals=CAN2_IVI_HMI_CustmiFun_Sta
  bus_selector8 : BusSelector  OutputSignals=CAN2_IVI_HMI_CustmiKEY_Sta
  bus_selector9 : BusSelector  OutputSignals=CAN2_IVI_LSEATvent_Cmd
  VHAL_IVICLBlowerYSta_pct : Outport
  VHAL_IVICLBlowerZSta_pct : Outport  Port=2
  VHAL_IVICRBlowerYSta_pct : Outport  Port=3
  VHAL_IVICRBlowerZSta_pct : Outport  Port=4
  VHAL_IVIDrBlowerModeSta_enum : Outport  Port=5
  VHAL_IVIDrBlowerYSta_pct : Outport  Port=6
  VHAL_IVIDrBlowerZSta_pct : Outport  Port=7
  VHAL_IVIHMICustmiFunSta_enum : Outport  Port=8
  VHAL_IVIHMICustmiKEYSta_enum : Outport  Port=9
  VHAL_IVILSEATventCmd_enum : Outport  Port=10
  VHAL_IVIMLFMostCmd_flg : Outport  Port=11
  VHAL_IVIMLFootLiftCmd_enum : Outport  Port=12
  VHAL_IVIMLNapModeCmd_flg : Outport  Port=13
  VHAL_IVIMLReclinerCmd_enum : Outport  Port=14
  VHAL_IVIMLRestoreCmd_flg : Outport  Port=15
  VHAL_IVIMLSEATventCmd_enum : Outport  Port=16
  VHAL_IVIMLSeatLiftCmd_enum : Outport  Port=17
  VHAL_IVIMLSldRestoreCmd_flg : Outport  Port=18
  VHAL_IVIMLSliderCmd_enum : Outport  Port=19
  VHAL_IVIMLZeroGravityCmd_flg : Outport  Port=20
  VHAL_IVIMRFMostCmd_flg : Outport  Port=21
  VHAL_IVIMRFootLiftCmd_enum : Outport  Port=22
  VHAL_IVIMRNapModeCmd_flg : Outport  Port=23
  VHAL_IVIMRReclinerCmd_enum : Outport  Port=24
  VHAL_IVIMRRestoreCmd_flg : Outport  Port=25
  VHAL_IVIMRSEATventCmd_enum : Outport  Port=26
  VHAL_IVIMRSeatLiftCmd_enum : Outport  Port=27
  VHAL_IVIMRSldRestoreCmd_flg : Outport  Port=28
  VHAL_IVIMRSliderCmd_enum : Outport  Port=29
  VHAL_IVIMRZeroGravityCmd_flg : Outport  Port=30
  VHAL_IVIPsBlowerModeSta_enum : Outport  Port=31
  VHAL_IVIPsBlowerYSta_pct : Outport  Port=32
  VHAL_IVIPsBlowerZSta_pct : Outport  Port=33
  VHAL_IVIRSEATventCmd_enum : Outport  Port=34
  VHAL_IVISnowModeCmd_flg : Outport  Port=35
  VHAL_IVIUserTakeOverAPSSta_flg : Outport  Port=36
  VHAL_IVIZon1WindDirSWReqSta_flg : Outport  Port=37
  wires:
  DT_CAN2_SG_IVI3/1 -> [DT_CAN2_SG_IVI3]
  [DT_CAN2_SG_IVI3] -> bus_selector/1
  bus_selector/1 -> IVICLBlowerYSta/1(IVI_CLBlower_Y_Sta)  "<CAN2_IVI_CLBlower_Y_Sta>"
  IVICLBlowerYSta/1(VHAL_IVICLBlowerYSta_pct) -> VHAL_IVICLBlowerYSta_pct/1
  [DT_CAN2_SG_IVI3] -> bus_selector1/1
  bus_selector1/1 -> IVICLBlowerZSta/1(IVI_CLBlower_Z_Sta)  "<CAN2_IVI_CLBlower_Z_Sta>"
  IVICLBlowerZSta/1(VHAL_IVICLBlowerZSta_pct) -> VHAL_IVICLBlowerZSta_pct/1
  [DT_CAN2_SG_IVI3] -> bus_selector2/1
  bus_selector2/1 -> IVICRBlowerYSta/1(IVI_CRBlower_Y_Sta)  "<CAN2_IVI_CRBlower_Y_Sta>"
  IVICRBlowerYSta/1(VHAL_IVICRBlowerYSta_pct) -> VHAL_IVICRBlowerYSta_pct/1
  [DT_CAN2_SG_IVI3] -> bus_selector3/1
  bus_selector3/1 -> IVICRBlowerZSta/1(IVI_CRBlower_Z_Sta)  "<CAN2_IVI_CRBlower_Z_Sta>"
  IVICRBlowerZSta/1(VHAL_IVICRBlowerZSta_pct) -> VHAL_IVICRBlowerZSta_pct/1
  [DT_CAN2_SG_IVI3] -> bus_selector4/1
  bus_selector4/1 -> IVIDrBlowerModeSta/1(IVI_DrBlower_Mode_Sta)  "<CAN2_IVI_DrBlower_Mode_Sta>"
  IVIDrBlowerModeSta/1(VHAL_IVIDrBlowerModeSta_enum) -> VHAL_IVIDrBlowerModeSta_enum/1
  [DT_CAN2_SG_IVI3] -> bus_selector5/1
  bus_selector5/1 -> IVIDrBlowerYSta/1(IVI_DrBlower_Y_Sta)  "<CAN2_IVI_DrBlower_Y_Sta>"
  IVIDrBlowerYSta/1(VHAL_IVIDrBlowerYSta_pct) -> VHAL_IVIDrBlowerYSta_pct/1
  [DT_CAN2_SG_IVI3] -> bus_selector6/1
  bus_selector6/1 -> IVIDrBlowerZSta/1(IVI_DrBlower_Z_Sta)  "<CAN2_IVI_DrBlower_Z_Sta>"
  IVIDrBlowerZSta/1(VHAL_IVIDrBlowerZSta_pct) -> VHAL_IVIDrBlowerZSta_pct/1
  [DT_CAN2_SG_IVI3] -> bus_selector7/1
  bus_selector7/1 -> IVIHMICustmiFunSta/1(IVI_HMI_CustmiFun_Sta)  "<CAN2_IVI_HMI_CustmiFun_Sta>"
  IVIHMICustmiFunSta/1(VHAL_IVIHMICustmiFunSta_enum) -> VHAL_IVIHMICustmiFunSta_enum/1
  [DT_CAN2_SG_IVI3] -> bus_selector8/1
  bus_selector8/1 -> IVIHMICustmiKEYSta/1(IVI_HMI_CustmiKEY_Sta)  "<CAN2_IVI_HMI_CustmiKEY_Sta>"
  IVIHMICustmiKEYSta/1(VHAL_IVIHMICustmiKEYSta_enum) -> VHAL_IVIHMICustmiKEYSta_enum/1
  [DT_CAN2_SG_IVI3] -> bus_selector9/1
  bus_selector9/1 -> IVILSEATventCmd/1(IVI_LSEATvent_Cmd)  "<CAN2_IVI_LSEATvent_Cmd>"
  IVILSEATventCmd/1(VHAL_IVILSEATventCmd_enum) -> VHAL_IVILSEATventCmd_enum/1
  [DT_CAN2_SG_IVI3] -> bus_selector10/1
  bus_selector10/1 -> IVIMLFMostCmd/1(IVI_MLFMost_Cmd)  "<CAN2_IVI_MLFMost_Cmd>"
  IVIMLFMostCmd/1(VHAL_IVIMLFMostCmd_flg) -> VHAL_IVIMLFMostCmd_flg/1
  [DT_CAN2_SG_IVI3] -> bus_selector11/1
  bus_selector11/1 -> IVIMLFootLiftCmd/1(IVI_MLFootLift_Cmd)  "<CAN2_IVI_MLFootLift_Cmd>"
  IVIMLFootLiftCmd/1(VHAL_IVIMLFootLiftCmd_enum) -> VHAL_IVIMLFootLiftCmd_enum/1
  [DT_CAN2_SG_IVI3] -> bus_selector12/1
  bus_selector12/1 -> IVIMLNapModeCmd/1(IVI_MLNapMode_Cmd)  "<CAN2_IVI_MLNapMode_Cmd>"
  IVIMLNapModeCmd/1(VHAL_IVIMLNapModeCmd_flg) -> VHAL_IVIMLNapModeCmd_flg/1
  [DT_CAN2_SG_IVI3] -> bus_selector13/1
  bus_selector13/1 -> IVIMLReclinerCmd/1(IVI_MLRecliner_Cmd)  "<CAN2_IVI_MLRecliner_Cmd>"
  IVIMLReclinerCmd/1(VHAL_IVIMLReclinerCmd_enum) -> VHAL_IVIMLReclinerCmd_enum/1
  [DT_CAN2_SG_IVI3] -> bus_selector14/1
  bus_selector14/1 -> IVIMLRestoreCmd/1(IVI_MLRestore_Cmd)  "<CAN2_IVI_MLRestore_Cmd>"
  IVIMLRestoreCmd/1(VHAL_IVIMLRestoreCmd_flg) -> VHAL_IVIMLRestoreCmd_flg/1
  [DT_CAN2_SG_IVI3] -> bus_selector15/1
  bus_selector15/1 -> IVIMLSEATventCmd/1(IVI_MLSEATvent_Cmd)  "<CAN2_IVI_MLSEATvent_Cmd>"
  IVIMLSEATventCmd/1(VHAL_IVIMLSEATventCmd_enum) -> VHAL_IVIMLSEATventCmd_enum/1
  [DT_CAN2_SG_IVI3] -> bus_selector16/1
  bus_selector16/1 -> IVIMLSeatLiftCmd/1(IVI_MLSeatLift_Cmd)  "<CAN2_IVI_MLSeatLift_Cmd>"
  IVIMLSeatLiftCmd/1(VHAL_IVIMLSeatLiftCmd_enum) -> VHAL_IVIMLSeatLiftCmd_enum/1
  [DT_CAN2_SG_IVI3] -> bus_selector17/1
  bus_selector17/1 -> IVIMLSldRestoreCmd/1(IVI_MLSldRestore_Cmd)  "<CAN2_IVI_MLSldRestore_Cmd>"
  IVIMLSldRestoreCmd/1(VHAL_IVIMLSldRestoreCmd_flg) -> VHAL_IVIMLSldRestoreCmd_flg/1
  [DT_CAN2_SG_IVI3] -> bus_selector18/1
  bus_selector18/1 -> IVIMLSliderCmd/1(IVI_MLSlider_Cmd)  "<CAN2_IVI_MLSlider_Cmd>"
  IVIMLSliderCmd/1(VHAL_IVIMLSliderCmd_enum) -> VHAL_IVIMLSliderCmd_enum/1
  [DT_CAN2_SG_IVI3] -> bus_selector19/1
  bus_selector19/1 -> IVIMLZeroGravityCmd/1(IVI_MLZeroGravity_Cmd)  "<CAN2_IVI_MLZeroGravity_Cmd>"
  IVIMLZeroGravityCmd/1(VHAL_IVIMLZeroGravityCmd_flg) -> VHAL_IVIMLZeroGravityCmd_flg/1
  [DT_CAN2_SG_IVI3] -> bus_selector20/1
  bus_selector20/1 -> IVIMRFMostCmd/1(IVI_MRFMost_Cmd)  "<CAN2_IVI_MRFMost_Cmd>"
  IVIMRFMostCmd/1(VHAL_IVIMRFMostCmd_flg) -> VHAL_IVIMRFMostCmd_flg/1
  [DT_CAN2_SG_IVI3] -> bus_selector21/1
  bus_selector21/1 -> IVIMRFootLiftCmd/1(IVI_MRFootLift_Cmd)  "<CAN2_IVI_MRFootLift_Cmd>"
  IVIMRFootLiftCmd/1(VHAL_IVIMRFootLiftCmd_enum) -> VHAL_IVIMRFootLiftCmd_enum/1
  [DT_CAN2_SG_IVI3] -> bus_selector22/1
  bus_selector22/1 -> IVIMRNapModeCmd/1(IVI_MRNapMode_Cmd)  "<CAN2_IVI_MRNapMode_Cmd>"
  IVIMRNapModeCmd/1(VHAL_IVIMRNapModeCmd_flg) -> VHAL_IVIMRNapModeCmd_flg/1
  [DT_CAN2_SG_IVI3] -> bus_selector23/1
  bus_selector23/1 -> IVIMRReclinerCmd/1(IVI_MRRecliner_Cmd)  "<CAN2_IVI_MRRecliner_Cmd>"
  IVIMRReclinerCmd/1(VHAL_IVIMRReclinerCmd_enum) -> VHAL_IVIMRReclinerCmd_enum/1
  [DT_CAN2_SG_IVI3] -> bus_selector24/1
  bus_selector24/1 -> IVIMRRestoreCmd/1(IVI_MRRestore_Cmd)  "<CAN2_IVI_MRRestore_Cmd>"
  IVIMRRestoreCmd/1(VHAL_IVIMRRestoreCmd_flg) -> VHAL_IVIMRRestoreCmd_flg/1
  [DT_CAN2_SG_IVI3] -> bus_selector25/1
  bus_selector25/1 -> IVIMRSEATventCmd/1(IVI_MRSEATvent_Cmd)  "<CAN2_IVI_MRSEATvent_Cmd>"
  IVIMRSEATventCmd/1(VHAL_IVIMRSEATventCmd_enum) -> VHAL_IVIMRSEATventCmd_enum/1
  [DT_CAN2_SG_IVI3] -> bus_selector26/1
  bus_selector26/1 -> IVIMRSeatLiftCmd/1(IVI_MRSeatLift_Cmd)  "<CAN2_IVI_MRSeatLift_Cmd>"
  IVIMRSeatLiftCmd/1(VHAL_IVIMRSeatLiftCmd_enum) -> VHAL_IVIMRSeatLiftCmd_enum/1
  [DT_CAN2_SG_IVI3] -> bus_selector27/1
  bus_selector27/1 -> IVIMRSldRestoreCmd/1(IVI_MRSldRestore_Cmd)  "<CAN2_IVI_MRSldRestore_Cmd>"
  IVIMRSldRestoreCmd/1(VHAL_IVIMRSldRestoreCmd_flg) -> VHAL_IVIMRSldRestoreCmd_flg/1
  [DT_CAN2_SG_IVI3] -> bus_selector28/1
  bus_selector28/1 -> IVIMRSliderCmd/1(IVI_MRSlider_Cmd)  "<CAN2_IVI_MRSlider_Cmd>"
  IVIMRSliderCmd/1(VHAL_IVIMRSliderCmd_enum) -> VHAL_IVIMRSliderCmd_enum/1
  [DT_CAN2_SG_IVI3] -> bus_selector29/1
  bus_selector29/1 -> IVIMRZeroGravityCmd/1(IVI_MRZeroGravity_Cmd)  "<CAN2_IVI_MRZeroGravity_Cmd>"
  IVIMRZeroGravityCmd/1(VHAL_IVIMRZeroGravityCmd_flg) -> VHAL_IVIMRZeroGravityCmd_flg/1
  [DT_CAN2_SG_IVI3] -> bus_selector30/1
  bus_selector30/1 -> IVIPsBlowerModeSta/1(IVI_PsBlower_Mode_Sta)  "<CAN2_IVI_PsBlower_Mode_Sta>"
  IVIPsBlowerModeSta/1(VHAL_IVIPsBlowerModeSta_enum) -> VHAL_IVIPsBlowerModeSta_enum/1
  [DT_CAN2_SG_IVI3] -> bus_selector31/1
  bus_selector31/1 -> IVIPsBlowerYSta/1(IVI_PsBlower_Y_Sta)  "<CAN2_IVI_PsBlower_Y_Sta>"
  IVIPsBlowerYSta/1(VHAL_IVIPsBlowerYSta_pct) -> VHAL_IVIPsBlowerYSta_pct/1
  [DT_CAN2_SG_IVI3] -> bus_selector32/1
  bus_selector32/1 -> IVIPsBlowerZSta/1(IVI_PsBlower_Z_Sta)  "<CAN2_IVI_PsBlower_Z_Sta>"
  IVIPsBlowerZSta/1(VHAL_IVIPsBlowerZSta_pct) -> VHAL_IVIPsBlowerZSta_pct/1
  [DT_CAN2_SG_IVI3] -> bus_selector33/1
  bus_selector33/1 -> IVIRSEATventCmd/1(IVI_RSEATvent_Cmd)  "<CAN2_IVI_RSEATvent_Cmd>"
  IVIRSEATventCmd/1(VHAL_IVIRSEATventCmd_enum) -> VHAL_IVIRSEATventCmd_enum/1
  [DT_CAN2_SG_IVI3] -> bus_selector34/1
  bus_selector34/1 -> IVISnowModeCmd/1(IVI_SnowMode_Cmd)  "<CAN2_IVI_SnowMode_Cmd>"
  IVISnowModeCmd/1(VHAL_IVISnowModeCmd_flg) -> VHAL_IVISnowModeCmd_flg/1
  [DT_CAN2_SG_IVI3] -> bus_selector35/1
  bus_selector35/1 -> IVIUserTakeOverAPSSta/1(IVI_UserTakeOver_APS_Sta)  "<CAN2_IVI_UserTakeOver_APS_Sta>"
  IVIUserTakeOverAPSSta/1(VHAL_IVIUserTakeOverAPSSta_flg) -> VHAL_IVIUserTakeOverAPSSta_flg/1
  [DT_CAN2_SG_IVI3] -> bus_selector36/1
  bus_selector36/1 -> IVIZon1WindDirSWReqSta/1(IVI_Zon1WindDirSWReq_Sta)  "<CAN2_IVI_Zon1WindDirSWReq_Sta>"
  IVIZon1WindDirSWReqSta/1(VHAL_IVIZon1WindDirSWReqSta_flg) -> VHAL_IVIZon1WindDirSWReqSta_flg/1

== system halin/HAL_IN/CAN2/METER1 ==
  DT_CAN2_SG_METER1 : Inport
  METERKPHCalcu : Subsystem
  ODOMETER : Subsystem
  bus_selector : BusSelector  OutputSignals=CAN2_METER_KPH_Calcu
  bus_selector1 : BusSelector  OutputSignals=CAN2_ODOMETER
  VHAL_METERKPHCalcu_kph : Outport
  VHAL_ODOMETER_km : Outport  Port=2
  wires:
  DT_CAN2_SG_METER1/1 -> [DT_CAN2_SG_METER1]
  [DT_CAN2_SG_METER1] -> bus_selector/1
  bus_selector/1 -> METERKPHCalcu/1(METER_KPH_Calcu)  "<CAN2_METER_KPH_Calcu>"
  METERKPHCalcu/1(VHAL_METERKPHCalcu_kph) -> VHAL_METERKPHCalcu_kph/1
  [DT_CAN2_SG_METER1] -> bus_selector1/1
  bus_selector1/1 -> ODOMETER/1(ODOMETER)  "<CAN2_ODOMETER>"
  ODOMETER/1(VHAL_ODOMETER_km) -> VHAL_ODOMETER_km/1

== system halin/HAL_IN/CAN2/VHAL_CANMsgInvalidHMI1_flg ==
  Cast To Boolean13 : DataTypeConversion  OutDataTypeStr=boolean
  Constant : Constant  Value=TRUE
  Latch13 : hcu_lib/Basic_Blocks/Latch
  Switch13 : Switch  Criteria=u2 ~= 0
  Unit Delay : UnitDelay  SampleTime=-1  HasFrameUpgradeWarning=on
  UnitConverter : DataTypeConversion  OutDataTypeStr=boolean
  Out : Outport
  wires:
  Constant/1 -> Switch13/3
  Unit Delay/1 -> Cast To Boolean13/1
  Cast To Boolean13/1 -> Switch13/1, Latch13/1
  Switch13/1 -> UnitConverter/1
  Latch13/1 -> Switch13/2
  UnitConverter/1 -> Unit Delay/1, Out/1  "VHAL_CANMsgInvalidHMI1_flg"

== system halin/HAL_IN/CAN2/VHAL_CANMsgInvalidIVI1_flg ==
  Cast To Boolean13 : DataTypeConversion  OutDataTypeStr=boolean
  Constant : Constant  Value=TRUE
  Latch13 : hcu_lib/Basic_Blocks/Latch
  Switch13 : Switch  Criteria=u2 ~= 0
  Unit Delay : UnitDelay  SampleTime=-1  HasFrameUpgradeWarning=on
  UnitConverter : DataTypeConversion  OutDataTypeStr=boolean
  Out : Outport
  wires:
  Constant/1 -> Switch13/3
  Unit Delay/1 -> Cast To Boolean13/1
  Cast To Boolean13/1 -> Switch13/1, Latch13/1
  Switch13/1 -> UnitConverter/1
  Latch13/1 -> Switch13/2
  UnitConverter/1 -> Unit Delay/1, Out/1  "VHAL_CANMsgInvalidIVI1_flg"

== system halin/HAL_IN/CAN2/VHAL_CANMsgInvalidIVI2_flg ==
  Cast To Boolean13 : DataTypeConversion  OutDataTypeStr=boolean
  Constant : Constant  Value=TRUE
  Latch13 : hcu_lib/Basic_Blocks/Latch
  Switch13 : Switch  Criteria=u2 ~= 0
  Unit Delay : UnitDelay  SampleTime=-1  HasFrameUpgradeWarning=on
  UnitConverter : DataTypeConversion  OutDataTypeStr=boolean
  Out : Outport
  wires:
  Constant/1 -> Switch13/3
  Unit Delay/1 -> Cast To Boolean13/1
  Cast To Boolean13/1 -> Switch13/1, Latch13/1
  Switch13/1 -> UnitConverter/1
  Latch13/1 -> Switch13/2
  UnitConverter/1 -> Unit Delay/1, Out/1  "VHAL_CANMsgInvalidIVI2_flg"

== system halin/HAL_IN/CAN2/VHAL_CANMsgInvalidIVI3_flg ==
  Cast To Boolean13 : DataTypeConversion  OutDataTypeStr=boolean
  Constant : Constant  Value=TRUE
  Latch13 : hcu_lib/Basic_Blocks/Latch
  Switch13 : Switch  Criteria=u2 ~= 0
  Unit Delay : UnitDelay  SampleTime=-1  HasFrameUpgradeWarning=on
  UnitConverter : DataTypeConversion  OutDataTypeStr=boolean
  Out : Outport
  wires:
  Constant/1 -> Switch13/3
  Unit Delay/1 -> Cast To Boolean13/1
  Cast To Boolean13/1 -> Switch13/1, Latch13/1
  Switch13/1 -> UnitConverter/1
  Latch13/1 -> Switch13/2
  UnitConverter/1 -> Unit Delay/1, Out/1  "VHAL_CANMsgInvalidIVI3_flg"
